simulink model "SlidingModeRobot_before_feedforard"  (R2015b)
settings: Solver=ode4  StartTime=0.0  StopTime=20  FixedStep=0.01  RelTol=1e-3
InitFcn:
  | Set_Parameter
values from neighbouring files (symbols this model uses):
  b = 0.1    [Set_Parameter_Single.m]
  J = [0.016,0.016,0.012,0.012,0.01,0.01,0.01]    [Set_Parameter_Single.m]
  K = 0.01    [Set_Parameter_Single.m]
  L = 0.5    [Set_Parameter_Single.m]
  R = 1    [Set_Parameter_Single.m]
undefined symbols (not defined in the file or in its folder): IniJointAngle
libraries: simulink x14
settings Model: Creator=User  LastModifiedBy=User

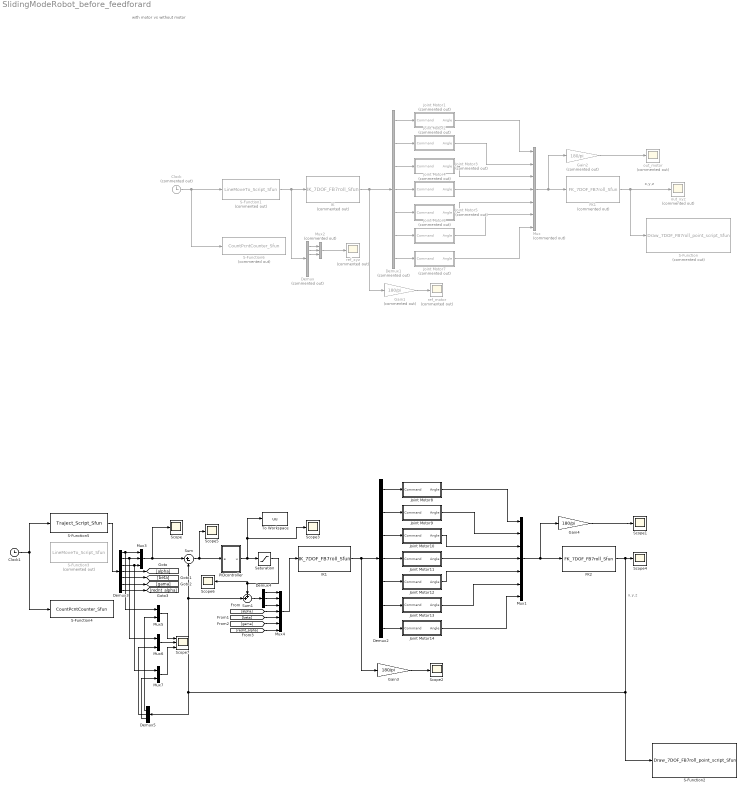
== system SlidingModeRobot_before_feedforard ==
  note: with motor vs without motor
  note: x,y,z
  note: x,y,z
  Clock : Clock  Commented=on
  Clock1 : Clock
  Demux : Demux  Commented=on  Outputs=7
  Demux1 : Demux  Commented=on  Outputs=7
  Demux2 : Demux  Outputs=7
  Demux3 : Demux  Outputs=7
  Demux4 : Demux  Outputs=3
  Demux5 : Demux  Outputs=3
  FK1 : S-Function  Commented=on  FunctionName=FK_7DOF_FB7roll_Sfun  SFunctionDeploymentMode=off  EnableBusSupport=off
  FK2 : S-Function  FunctionName=FK_7DOF_FB7roll_Sfun  SFunctionDeploymentMode=off  EnableBusSupport=off
  Gain1 : Gain  Commented=on  Gain=180/pi
  Gain2 : Gain  Commented=on  Gain=180/pi
  Gain3 : Gain  Gain=180/pi
  Gain4 : Gain  Gain=180/pi
  IK : S-Function  Commented=on  FunctionName=IK_7DOF_FB7roll_Sfun  SFunctionDeploymentMode=off  EnableBusSupport=off
  IK1 : S-Function  FunctionName=IK_7DOF_FB7roll_Sfun  SFunctionDeploymentMode=off  EnableBusSupport=off
  Joint Motor1 : Subsystem  Commented=on
  Joint Motor10 : Subsystem
  Joint Motor11 : Subsystem
  Joint Motor12 : Subsystem
  Joint Motor13 : Subsystem
  Joint Motor14 : Subsystem
  Joint Motor2 : Subsystem  Commented=on
  Joint Motor3 : Subsystem  Commented=on
  Joint Motor4 : Subsystem  Commented=on
  Joint Motor5 : Subsystem  Commented=on
  Joint Motor6 : Subsystem  Commented=on
  Joint Motor7 : Subsystem  Commented=on
  Joint Motor8 : Subsystem
  Joint Motor9 : Subsystem
  Mux : Mux  Commented=on  Inputs=7
  Mux1 : Mux  Inputs=7
  Mux2 : Mux  Commented=on  Inputs=3
  Mux3 : Mux  Inputs=3
  Mux4 : Mux  Inputs=7
  Mux5 : Mux  Inputs=2
  Mux6 : Mux  Inputs=2
  Mux7 : Mux  Inputs=2
  PIDcontroller : Subsystem
  S-Function : S-Function  Commented=on  FunctionName=Draw_7DOF_FB7roll_point_script_Sfun  SFunctionDeploymentMode=off  EnableBusSupport=off
  S-Function1 : S-Function  Commented=on  FunctionName=LineMoveTo_Script_Sfun  SFunctionDeploymentMode=off  EnableBusSupport=off
  S-Function2 : S-Function  FunctionName=Draw_7DOF_FB7roll_point_script_Sfun  SFunctionDeploymentMode=off  EnableBusSupport=off
  S-Function3 : S-Function  Commented=on  FunctionName=LineMoveTo_Script_Sfun  SFunctionDeploymentMode=off  EnableBusSupport=off
  S-Function4 : S-Function  FunctionName=CountPcntCounter_Sfun  SFunctionDeploymentMode=off  EnableBusSupport=off
  S-Function5 : S-Function  FunctionName=Traject_Script_Sfun  SFunctionDeploymentMode=off  EnableBusSupport=off
  S-Function6 : S-Function  Commented=on  FunctionName=CountPcntCounter_Sfun  SFunctionDeploymentMode=off  EnableBusSupport=off
  Saturation : Saturate  UpperLimit=50  LowerLimit=-50
  Scope{,1..6} (7 alike) : Scope
  Scope7 : Scope  NumInputPorts=3
  Sum : Sum  Inputs=|+-
  Sum1 : Sum  Inputs=++|
  To Workspace : ToWorkspace  VariableName=uu  SaveFormat=Timeseries  SampleTime=-1
  out_motor : Scope  Commented=on
  out_xyz : Scope  Commented=on
  ref_motor : Scope  Commented=on
  ref_xyz : Scope  Commented=on
  wires:
  Joint Motor3/1(Angle) -> Mux/3
  Joint Motor1/1(Angle) -> Mux/1
  Joint Motor2/1(Angle) -> Mux/2
  Joint Motor4/1(Angle) -> Mux/4
  Joint Motor5/1(Angle) -> Mux/5
  Joint Motor6/1(Angle) -> Mux/6
  Joint Motor7/1(Angle) -> Mux/7
  S-Function1/1 -> Demux/1, IK/1
  Gain1/1 -> ref_motor/1
  FK1/1 -> S-Function/1, out_xyz/1
  Gain2/1 -> out_motor/1
  Demux1/7 -> Joint Motor7/1(Command)
  Demux1/6 -> Joint Motor6/1(Command)
  Demux1/5 -> Joint Motor5/1(Command)
  Demux1/4 -> Joint Motor4/1(Command)
  Demux1/1 -> Joint Motor1/1(Command)
  Demux1/2 -> Joint Motor2/1(Command)
  Demux1/3 -> Joint Motor3/1(Command)
  IK/1 -> Demux1/1, Gain1/1
  Clock/1 -> S-Function6/1, S-Function1/1
  Mux/1 -> Gain2/1, FK1/1
  Joint Motor10/1(Angle) -> Mux1/3
  Joint Motor8/1(Angle) -> Mux1/1
  Joint Motor9/1(Angle) -> Mux1/2
  Joint Motor11/1(Angle) -> Mux1/4
  Joint Motor12/1(Angle) -> Mux1/5
  Joint Motor13/1(Angle) -> Mux1/6
  Joint Motor14/1(Angle) -> Mux1/7
  Gain3/1 -> Scope2/1
  FK2/1 -> Scope4/1, S-Function2/1, Sum1/2, Sum/2, Demux5/1
  Gain4/1 -> Scope1/1
  Demux2/7 -> Joint Motor14/1(Command)
  Demux2/6 -> Joint Motor13/1(Command)
  Demux2/5 -> Joint Motor12/1(Command)
  Demux2/4 -> Joint Motor11/1(Command)
  Demux2/1 -> Joint Motor8/1(Command)
  Demux2/2 -> Joint Motor9/1(Command)
  Demux2/3 -> Joint Motor10/1(Command)
  IK1/1 -> Demux2/1, Gain3/1
  Clock1/1 -> S-Function5/1, S-Function4/1
  Mux1/1 -> Gain4/1, FK2/1
  Sum/1 -> Scope5/1, PIDcontroller/1(e)
  Demux/1 -> Mux2/1
  Demux/2 -> Mux2/2
  Demux/3 -> Mux2/3
  Mux2/1 -> ref_xyz/1
  Demux3/1 -> Mux3/1, Mux5/1
  Demux3/2 -> Mux3/2, Mux6/1
  Demux3/3 -> Mux7/1, Mux3/3
  Demux3/4 -> [alpha]
  Demux3/5 -> [beta]
  Demux3/6 -> [gama]
  [gama] -> Mux4/6
  [beta] -> Mux4/5
  [alpha] -> Mux4/4
  Demux4/1 -> Mux4/1
  Demux4/2 -> Mux4/2
  Demux4/3 -> Mux4/3
  PIDcontroller/1(u) -> Scope3/1, To Workspace/1, Saturation/1
  Mux4/1 -> IK1/1
  Demux3/7 -> [rednt_alpha]
  [rednt_alpha] -> Mux4/7
  Sum1/1 -> Demux4/1
  Saturation/1 -> Scope6/1, Sum1/1
  S-Function5/1 -> Demux3/1
  Mux3/1 -> Sum/1, Scope/1
  Demux5/1 -> Mux5/2
  Demux5/2 -> Mux6/2
  Demux5/3 -> Mux7/2
  Mux6/1 -> Scope7/2
  Mux5/1 -> Scope7/1
  Mux7/1 -> Scope7/3

== system SlidingModeRobot_before_feedforard/Joint Motor1 ==
  Command : Inport
  Constant : Constant  Value=IniJointAngle(1)
  DC motor : Subsystem
  Gain : Gain  Gain=30
  Integrator : Integrator  InitialConditionSource=external
  PID Controller : simulink/Continuous/PID Controller  Controller=PID  TimeDomain=Continuous-time  SampleTime=-1  IntegratorMethod=Forward Euler  FilterMethod=Forward Euler  Form=Parallel  UseFilter=on  ControllerParametersSource=internal  P=20  I=0  D=20  N=0  InitialConditionSource=internal  InitialConditionForIntegrator=0  InitialConditionForFilter=0  ExternalReset=none  LimitOutput=off  UpperSaturationLimit=inf  LowerSaturationLimit=-inf  LinearizeAsGain=on  AntiWindupMode=none  Kb=1  TrackingMode=off  Kt=1  PParamMin=[]  PParamMax=[]  IParamMin=[]  IParamMax=[]  DParamMin=[]  DParamMax=[]  NParamMin=[]  NParamMax=[]  KbParamMin=[]  KbParamMax=[]  KtParamMin=[]  KtParamMax=[]  POutMin=[]  POutMax=[]  IOutMin=[]  IOutMax=[]  DOutMin=[]  DOutMax=[]  NOutMin=[]  NOutMax=[]  KbOutMin=[]  KbOutMax=[]  KtOutMin=[]  KtOutMax=[]  IntegratorOutMin=[]  IntegratorOutMax=[]  FilterOutMin=[]  FilterOutMax=[]  SumOutMin=[]  SumOutMax=[]  SumI1OutMin=[]  SumI1OutMax=[]  SumI2OutMin=[]  SumI2OutMax=[]  SumI3OutMin=[]  SumI3OutMax=[]  SumDOutMin=[]  SumDOutMax=[]  SaturationOutMin=[]  SaturationOutMax=[]  IntegratorContinuousStateAttributes=''  IntegratorStateMustResolveToSignalObject=off  IntegratorRTWStateStorageClass=Auto  FilterContinuousStateAttributes=''  FilterStateMustResolveToSignalObject=off  FilterRTWStateStorageClass=Auto  DifferentiatorICPrevScaledInput=0  DifferentiatorOutMin=[]  DifferentiatorOutMax=[]
  Sum : Sum  Inputs=|+-
  Sum1 : Sum  Inputs=|+-
  Angle : Outport
  wires:
  Sum/1 -> PID Controller/1
  PID Controller/1 -> DC motor/1(Voltage)
  DC motor/1(Speed) -> Sum/2, Integrator/1
  Integrator/1 -> Angle/1, Sum1/2
  Command/1 -> Sum1/1
  Sum1/1 -> Gain/1
  Gain/1 -> Sum/1
  Constant/1 -> Integrator/2

== system SlidingModeRobot_before_feedforard/Joint Motor10 ==
  Command : Inport
  Constant : Constant  Value=IniJointAngle(3)
  DC motor : Subsystem
  Gain : Gain  Gain=2
  Integrator : Integrator  InitialConditionSource=external
  PID Controller : simulink/Continuous/PID Controller  Controller=PID  TimeDomain=Continuous-time  SampleTime=-1  IntegratorMethod=Forward Euler  FilterMethod=Forward Euler  Form=Parallel  UseFilter=on  ControllerParametersSource=internal  P=20  I=0  D=20  N=0  InitialConditionSource=internal  InitialConditionForIntegrator=0  InitialConditionForFilter=0  ExternalReset=none  LimitOutput=off  UpperSaturationLimit=inf  LowerSaturationLimit=-inf  LinearizeAsGain=on  AntiWindupMode=none  Kb=1  TrackingMode=off  Kt=1  PParamMin=[]  PParamMax=[]  IParamMin=[]  IParamMax=[]  DParamMin=[]  DParamMax=[]  NParamMin=[]  NParamMax=[]  KbParamMin=[]  KbParamMax=[]  KtParamMin=[]  KtParamMax=[]  POutMin=[]  POutMax=[]  IOutMin=[]  IOutMax=[]  DOutMin=[]  DOutMax=[]  NOutMin=[]  NOutMax=[]  KbOutMin=[]  KbOutMax=[]  KtOutMin=[]  KtOutMax=[]  IntegratorOutMin=[]  IntegratorOutMax=[]  FilterOutMin=[]  FilterOutMax=[]  SumOutMin=[]  SumOutMax=[]  SumI1OutMin=[]  SumI1OutMax=[]  SumI2OutMin=[]  SumI2OutMax=[]  SumI3OutMin=[]  SumI3OutMax=[]  SumDOutMin=[]  SumDOutMax=[]  SaturationOutMin=[]  SaturationOutMax=[]  IntegratorContinuousStateAttributes=''  IntegratorStateMustResolveToSignalObject=off  IntegratorRTWStateStorageClass=Auto  FilterContinuousStateAttributes=''  FilterStateMustResolveToSignalObject=off  FilterRTWStateStorageClass=Auto  DifferentiatorICPrevScaledInput=0  DifferentiatorOutMin=[]  DifferentiatorOutMax=[]
  Sum : Sum  Inputs=|+-
  Sum1 : Sum  Inputs=|+-
  Angle : Outport
  wires:
  Sum/1 -> PID Controller/1
  PID Controller/1 -> DC motor/1(Voltage)
  DC motor/1(Speed) -> Sum/2, Integrator/1
  Integrator/1 -> Angle/1, Sum1/2
  Command/1 -> Sum1/1
  Sum1/1 -> Gain/1
  Gain/1 -> Sum/1
  Constant/1 -> Integrator/2

== system SlidingModeRobot_before_feedforard/Joint Motor11 ==
  Command : Inport
  Constant : Constant  Value=IniJointAngle(4)
  DC motor : Subsystem
  Gain : Gain  Gain=2
  Integrator : Integrator  InitialConditionSource=external
  PID Controller : simulink/Continuous/PID Controller  Controller=PID  TimeDomain=Continuous-time  SampleTime=-1  IntegratorMethod=Forward Euler  FilterMethod=Forward Euler  Form=Parallel  UseFilter=on  ControllerParametersSource=internal  P=20  I=0  D=20  N=0  InitialConditionSource=internal  InitialConditionForIntegrator=0  InitialConditionForFilter=0  ExternalReset=none  LimitOutput=off  UpperSaturationLimit=inf  LowerSaturationLimit=-inf  LinearizeAsGain=on  AntiWindupMode=none  Kb=1  TrackingMode=off  Kt=1  PParamMin=[]  PParamMax=[]  IParamMin=[]  IParamMax=[]  DParamMin=[]  DParamMax=[]  NParamMin=[]  NParamMax=[]  KbParamMin=[]  KbParamMax=[]  KtParamMin=[]  KtParamMax=[]  POutMin=[]  POutMax=[]  IOutMin=[]  IOutMax=[]  DOutMin=[]  DOutMax=[]  NOutMin=[]  NOutMax=[]  KbOutMin=[]  KbOutMax=[]  KtOutMin=[]  KtOutMax=[]  IntegratorOutMin=[]  IntegratorOutMax=[]  FilterOutMin=[]  FilterOutMax=[]  SumOutMin=[]  SumOutMax=[]  SumI1OutMin=[]  SumI1OutMax=[]  SumI2OutMin=[]  SumI2OutMax=[]  SumI3OutMin=[]  SumI3OutMax=[]  SumDOutMin=[]  SumDOutMax=[]  SaturationOutMin=[]  SaturationOutMax=[]  IntegratorContinuousStateAttributes=''  IntegratorStateMustResolveToSignalObject=off  IntegratorRTWStateStorageClass=Auto  FilterContinuousStateAttributes=''  FilterStateMustResolveToSignalObject=off  FilterRTWStateStorageClass=Auto  DifferentiatorICPrevScaledInput=0  DifferentiatorOutMin=[]  DifferentiatorOutMax=[]
  Sum : Sum  Inputs=|+-
  Sum1 : Sum  Inputs=|+-
  Angle : Outport
  wires:
  Sum/1 -> PID Controller/1
  PID Controller/1 -> DC motor/1(Voltage)
  DC motor/1(Speed) -> Sum/2, Integrator/1
  Integrator/1 -> Angle/1, Sum1/2
  Command/1 -> Sum1/1
  Sum1/1 -> Gain/1
  Gain/1 -> Sum/1
  Constant/1 -> Integrator/2

== system SlidingModeRobot_before_feedforard/Joint Motor12 ==
  Command : Inport
  Constant : Constant  Value=IniJointAngle(5)
  DC motor : Subsystem
  Gain : Gain  Gain=2
  Integrator : Integrator  InitialConditionSource=external
  PID Controller : simulink/Continuous/PID Controller  Controller=PID  TimeDomain=Continuous-time  SampleTime=-1  IntegratorMethod=Forward Euler  FilterMethod=Forward Euler  Form=Parallel  UseFilter=on  ControllerParametersSource=internal  P=20  I=0  D=20  N=0  InitialConditionSource=internal  InitialConditionForIntegrator=0  InitialConditionForFilter=0  ExternalReset=none  LimitOutput=off  UpperSaturationLimit=inf  LowerSaturationLimit=-inf  LinearizeAsGain=on  AntiWindupMode=none  Kb=1  TrackingMode=off  Kt=1  PParamMin=[]  PParamMax=[]  IParamMin=[]  IParamMax=[]  DParamMin=[]  DParamMax=[]  NParamMin=[]  NParamMax=[]  KbParamMin=[]  KbParamMax=[]  KtParamMin=[]  KtParamMax=[]  POutMin=[]  POutMax=[]  IOutMin=[]  IOutMax=[]  DOutMin=[]  DOutMax=[]  NOutMin=[]  NOutMax=[]  KbOutMin=[]  KbOutMax=[]  KtOutMin=[]  KtOutMax=[]  IntegratorOutMin=[]  IntegratorOutMax=[]  FilterOutMin=[]  FilterOutMax=[]  SumOutMin=[]  SumOutMax=[]  SumI1OutMin=[]  SumI1OutMax=[]  SumI2OutMin=[]  SumI2OutMax=[]  SumI3OutMin=[]  SumI3OutMax=[]  SumDOutMin=[]  SumDOutMax=[]  SaturationOutMin=[]  SaturationOutMax=[]  IntegratorContinuousStateAttributes=''  IntegratorStateMustResolveToSignalObject=off  IntegratorRTWStateStorageClass=Auto  FilterContinuousStateAttributes=''  FilterStateMustResolveToSignalObject=off  FilterRTWStateStorageClass=Auto  DifferentiatorICPrevScaledInput=0  DifferentiatorOutMin=[]  DifferentiatorOutMax=[]
  Sum : Sum  Inputs=|+-
  Sum1 : Sum  Inputs=|+-
  Angle : Outport
  wires:
  Sum/1 -> PID Controller/1
  PID Controller/1 -> DC motor/1(Voltage)
  DC motor/1(Speed) -> Sum/2, Integrator/1
  Integrator/1 -> Angle/1, Sum1/2
  Command/1 -> Sum1/1
  Sum1/1 -> Gain/1
  Gain/1 -> Sum/1
  Constant/1 -> Integrator/2

== system SlidingModeRobot_before_feedforard/Joint Motor13 ==
  Command : Inport
  Constant : Constant  Value=IniJointAngle(6)
  DC motor : Subsystem
  Gain : Gain  Gain=2
  Integrator : Integrator  InitialConditionSource=external
  PID Controller : simulink/Continuous/PID Controller  Controller=PID  TimeDomain=Continuous-time  SampleTime=-1  IntegratorMethod=Forward Euler  FilterMethod=Forward Euler  Form=Parallel  UseFilter=on  ControllerParametersSource=internal  P=20  I=0  D=20  N=0  InitialConditionSource=internal  InitialConditionForIntegrator=0  InitialConditionForFilter=0  ExternalReset=none  LimitOutput=off  UpperSaturationLimit=inf  LowerSaturationLimit=-inf  LinearizeAsGain=on  AntiWindupMode=none  Kb=1  TrackingMode=off  Kt=1  PParamMin=[]  PParamMax=[]  IParamMin=[]  IParamMax=[]  DParamMin=[]  DParamMax=[]  NParamMin=[]  NParamMax=[]  KbParamMin=[]  KbParamMax=[]  KtParamMin=[]  KtParamMax=[]  POutMin=[]  POutMax=[]  IOutMin=[]  IOutMax=[]  DOutMin=[]  DOutMax=[]  NOutMin=[]  NOutMax=[]  KbOutMin=[]  KbOutMax=[]  KtOutMin=[]  KtOutMax=[]  IntegratorOutMin=[]  IntegratorOutMax=[]  FilterOutMin=[]  FilterOutMax=[]  SumOutMin=[]  SumOutMax=[]  SumI1OutMin=[]  SumI1OutMax=[]  SumI2OutMin=[]  SumI2OutMax=[]  SumI3OutMin=[]  SumI3OutMax=[]  SumDOutMin=[]  SumDOutMax=[]  SaturationOutMin=[]  SaturationOutMax=[]  IntegratorContinuousStateAttributes=''  IntegratorStateMustResolveToSignalObject=off  IntegratorRTWStateStorageClass=Auto  FilterContinuousStateAttributes=''  FilterStateMustResolveToSignalObject=off  FilterRTWStateStorageClass=Auto  DifferentiatorICPrevScaledInput=0  DifferentiatorOutMin=[]  DifferentiatorOutMax=[]
  Sum : Sum  Inputs=|+-
  Sum1 : Sum  Inputs=|+-
  Angle : Outport
  wires:
  Sum/1 -> PID Controller/1
  PID Controller/1 -> DC motor/1(Voltage)
  DC motor/1(Speed) -> Sum/2, Integrator/1
  Integrator/1 -> Angle/1, Sum1/2
  Command/1 -> Sum1/1
  Sum1/1 -> Gain/1
  Gain/1 -> Sum/1
  Constant/1 -> Integrator/2

== system SlidingModeRobot_before_feedforard/Joint Motor14 ==
  Command : Inport
  Constant : Constant  Value=IniJointAngle(7)
  DC motor : Subsystem
  Gain : Gain  Gain=2
  Integrator : Integrator  InitialConditionSource=external
  PID Controller : simulink/Continuous/PID Controller  Controller=PID  TimeDomain=Continuous-time  SampleTime=-1  IntegratorMethod=Forward Euler  FilterMethod=Forward Euler  Form=Parallel  UseFilter=on  ControllerParametersSource=internal  P=20  I=0  D=20  N=0  InitialConditionSource=internal  InitialConditionForIntegrator=0  InitialConditionForFilter=0  ExternalReset=none  LimitOutput=off  UpperSaturationLimit=inf  LowerSaturationLimit=-inf  LinearizeAsGain=on  AntiWindupMode=none  Kb=1  TrackingMode=off  Kt=1  PParamMin=[]  PParamMax=[]  IParamMin=[]  IParamMax=[]  DParamMin=[]  DParamMax=[]  NParamMin=[]  NParamMax=[]  KbParamMin=[]  KbParamMax=[]  KtParamMin=[]  KtParamMax=[]  POutMin=[]  POutMax=[]  IOutMin=[]  IOutMax=[]  DOutMin=[]  DOutMax=[]  NOutMin=[]  NOutMax=[]  KbOutMin=[]  KbOutMax=[]  KtOutMin=[]  KtOutMax=[]  IntegratorOutMin=[]  IntegratorOutMax=[]  FilterOutMin=[]  FilterOutMax=[]  SumOutMin=[]  SumOutMax=[]  SumI1OutMin=[]  SumI1OutMax=[]  SumI2OutMin=[]  SumI2OutMax=[]  SumI3OutMin=[]  SumI3OutMax=[]  SumDOutMin=[]  SumDOutMax=[]  SaturationOutMin=[]  SaturationOutMax=[]  IntegratorContinuousStateAttributes=''  IntegratorStateMustResolveToSignalObject=off  IntegratorRTWStateStorageClass=Auto  FilterContinuousStateAttributes=''  FilterStateMustResolveToSignalObject=off  FilterRTWStateStorageClass=Auto  DifferentiatorICPrevScaledInput=0  DifferentiatorOutMin=[]  DifferentiatorOutMax=[]
  Sum : Sum  Inputs=|+-
  Sum1 : Sum  Inputs=|+-
  Angle : Outport
  wires:
  Sum/1 -> PID Controller/1
  PID Controller/1 -> DC motor/1(Voltage)
  DC motor/1(Speed) -> Sum/2, Integrator/1
  Integrator/1 -> Angle/1, Sum1/2
  Command/1 -> Sum1/1
  Sum1/1 -> Gain/1
  Gain/1 -> Sum/1
  Constant/1 -> Integrator/2

== system SlidingModeRobot_before_feedforard/Joint Motor2 ==
  Command : Inport
  Constant : Constant  Value=IniJointAngle(2)
  DC motor : Subsystem
  Gain : Gain  Gain=32
  Integrator : Integrator  InitialConditionSource=external
  PID Controller : simulink/Continuous/PID Controller  Controller=PID  TimeDomain=Continuous-time  SampleTime=-1  IntegratorMethod=Forward Euler  FilterMethod=Forward Euler  Form=Parallel  UseFilter=on  ControllerParametersSource=internal  P=20  I=0  D=20  N=0  InitialConditionSource=internal  InitialConditionForIntegrator=0  InitialConditionForFilter=0  ExternalReset=none  LimitOutput=off  UpperSaturationLimit=inf  LowerSaturationLimit=-inf  LinearizeAsGain=on  AntiWindupMode=none  Kb=1  TrackingMode=off  Kt=1  PParamMin=[]  PParamMax=[]  IParamMin=[]  IParamMax=[]  DParamMin=[]  DParamMax=[]  NParamMin=[]  NParamMax=[]  KbParamMin=[]  KbParamMax=[]  KtParamMin=[]  KtParamMax=[]  POutMin=[]  POutMax=[]  IOutMin=[]  IOutMax=[]  DOutMin=[]  DOutMax=[]  NOutMin=[]  NOutMax=[]  KbOutMin=[]  KbOutMax=[]  KtOutMin=[]  KtOutMax=[]  IntegratorOutMin=[]  IntegratorOutMax=[]  FilterOutMin=[]  FilterOutMax=[]  SumOutMin=[]  SumOutMax=[]  SumI1OutMin=[]  SumI1OutMax=[]  SumI2OutMin=[]  SumI2OutMax=[]  SumI3OutMin=[]  SumI3OutMax=[]  SumDOutMin=[]  SumDOutMax=[]  SaturationOutMin=[]  SaturationOutMax=[]  IntegratorContinuousStateAttributes=''  IntegratorStateMustResolveToSignalObject=off  IntegratorRTWStateStorageClass=Auto  FilterContinuousStateAttributes=''  FilterStateMustResolveToSignalObject=off  FilterRTWStateStorageClass=Auto  DifferentiatorICPrevScaledInput=0  DifferentiatorOutMin=[]  DifferentiatorOutMax=[]
  Sum : Sum  Inputs=|+-
  Sum1 : Sum  Inputs=|+-
  Angle : Outport
  wires:
  Sum/1 -> PID Controller/1
  PID Controller/1 -> DC motor/1(Voltage)
  DC motor/1(Speed) -> Sum/2, Integrator/1
  Integrator/1 -> Angle/1, Sum1/2
  Command/1 -> Sum1/1
  Sum1/1 -> Gain/1
  Gain/1 -> Sum/1
  Constant/1 -> Integrator/2

== system SlidingModeRobot_before_feedforard/Joint Motor3 ==
  Command : Inport
  Constant : Constant  Value=IniJointAngle(3)
  DC motor : Subsystem
  Gain : Gain  Gain=30
  Integrator : Integrator  InitialConditionSource=external
  PID Controller : simulink/Continuous/PID Controller  Controller=PID  TimeDomain=Continuous-time  SampleTime=-1  IntegratorMethod=Forward Euler  FilterMethod=Forward Euler  Form=Parallel  UseFilter=on  ControllerParametersSource=internal  P=20  I=0  D=20  N=0  InitialConditionSource=internal  InitialConditionForIntegrator=0  InitialConditionForFilter=0  ExternalReset=none  LimitOutput=off  UpperSaturationLimit=inf  LowerSaturationLimit=-inf  LinearizeAsGain=on  AntiWindupMode=none  Kb=1  TrackingMode=off  Kt=1  PParamMin=[]  PParamMax=[]  IParamMin=[]  IParamMax=[]  DParamMin=[]  DParamMax=[]  NParamMin=[]  NParamMax=[]  KbParamMin=[]  KbParamMax=[]  KtParamMin=[]  KtParamMax=[]  POutMin=[]  POutMax=[]  IOutMin=[]  IOutMax=[]  DOutMin=[]  DOutMax=[]  NOutMin=[]  NOutMax=[]  KbOutMin=[]  KbOutMax=[]  KtOutMin=[]  KtOutMax=[]  IntegratorOutMin=[]  IntegratorOutMax=[]  FilterOutMin=[]  FilterOutMax=[]  SumOutMin=[]  SumOutMax=[]  SumI1OutMin=[]  SumI1OutMax=[]  SumI2OutMin=[]  SumI2OutMax=[]  SumI3OutMin=[]  SumI3OutMax=[]  SumDOutMin=[]  SumDOutMax=[]  SaturationOutMin=[]  SaturationOutMax=[]  IntegratorContinuousStateAttributes=''  IntegratorStateMustResolveToSignalObject=off  IntegratorRTWStateStorageClass=Auto  FilterContinuousStateAttributes=''  FilterStateMustResolveToSignalObject=off  FilterRTWStateStorageClass=Auto  DifferentiatorICPrevScaledInput=0  DifferentiatorOutMin=[]  DifferentiatorOutMax=[]
  Sum : Sum  Inputs=|+-
  Sum1 : Sum  Inputs=|+-
  Angle : Outport
  wires:
  Sum/1 -> PID Controller/1
  PID Controller/1 -> DC motor/1(Voltage)
  DC motor/1(Speed) -> Sum/2, Integrator/1
  Integrator/1 -> Angle/1, Sum1/2
  Command/1 -> Sum1/1
  Sum1/1 -> Gain/1
  Gain/1 -> Sum/1
  Constant/1 -> Integrator/2

== system SlidingModeRobot_before_feedforard/Joint Motor4 ==
  Command : Inport
  Constant : Constant  Value=IniJointAngle(4)
  DC motor : Subsystem
  Gain : Gain  Gain=10
  Integrator : Integrator  InitialConditionSource=external
  PID Controller : simulink/Continuous/PID Controller  Controller=PID  TimeDomain=Continuous-time  SampleTime=-1  IntegratorMethod=Forward Euler  FilterMethod=Forward Euler  Form=Parallel  UseFilter=on  ControllerParametersSource=internal  P=20  I=0  D=20  N=0  InitialConditionSource=internal  InitialConditionForIntegrator=0  InitialConditionForFilter=0  ExternalReset=none  LimitOutput=off  UpperSaturationLimit=inf  LowerSaturationLimit=-inf  LinearizeAsGain=on  AntiWindupMode=none  Kb=1  TrackingMode=off  Kt=1  PParamMin=[]  PParamMax=[]  IParamMin=[]  IParamMax=[]  DParamMin=[]  DParamMax=[]  NParamMin=[]  NParamMax=[]  KbParamMin=[]  KbParamMax=[]  KtParamMin=[]  KtParamMax=[]  POutMin=[]  POutMax=[]  IOutMin=[]  IOutMax=[]  DOutMin=[]  DOutMax=[]  NOutMin=[]  NOutMax=[]  KbOutMin=[]  KbOutMax=[]  KtOutMin=[]  KtOutMax=[]  IntegratorOutMin=[]  IntegratorOutMax=[]  FilterOutMin=[]  FilterOutMax=[]  SumOutMin=[]  SumOutMax=[]  SumI1OutMin=[]  SumI1OutMax=[]  SumI2OutMin=[]  SumI2OutMax=[]  SumI3OutMin=[]  SumI3OutMax=[]  SumDOutMin=[]  SumDOutMax=[]  SaturationOutMin=[]  SaturationOutMax=[]  IntegratorContinuousStateAttributes=''  IntegratorStateMustResolveToSignalObject=off  IntegratorRTWStateStorageClass=Auto  FilterContinuousStateAttributes=''  FilterStateMustResolveToSignalObject=off  FilterRTWStateStorageClass=Auto  DifferentiatorICPrevScaledInput=0  DifferentiatorOutMin=[]  DifferentiatorOutMax=[]
  Sum : Sum  Inputs=|+-
  Sum1 : Sum  Inputs=|+-
  Angle : Outport
  wires:
  Sum/1 -> PID Controller/1
  PID Controller/1 -> DC motor/1(Voltage)
  DC motor/1(Speed) -> Sum/2, Integrator/1
  Integrator/1 -> Angle/1, Sum1/2
  Command/1 -> Sum1/1
  Sum1/1 -> Gain/1
  Gain/1 -> Sum/1
  Constant/1 -> Integrator/2

== system SlidingModeRobot_before_feedforard/Joint Motor5 ==
  Command : Inport
  Constant : Constant  Value=IniJointAngle(5)
  DC motor : Subsystem
  Gain : Gain  Gain=2
  Integrator : Integrator  InitialConditionSource=external
  PID Controller : simulink/Continuous/PID Controller  Controller=PID  TimeDomain=Continuous-time  SampleTime=-1  IntegratorMethod=Forward Euler  FilterMethod=Forward Euler  Form=Parallel  UseFilter=on  ControllerParametersSource=internal  P=20  I=0  D=20  N=0  InitialConditionSource=internal  InitialConditionForIntegrator=0  InitialConditionForFilter=0  ExternalReset=none  LimitOutput=off  UpperSaturationLimit=inf  LowerSaturationLimit=-inf  LinearizeAsGain=on  AntiWindupMode=none  Kb=1  TrackingMode=off  Kt=1  PParamMin=[]  PParamMax=[]  IParamMin=[]  IParamMax=[]  DParamMin=[]  DParamMax=[]  NParamMin=[]  NParamMax=[]  KbParamMin=[]  KbParamMax=[]  KtParamMin=[]  KtParamMax=[]  POutMin=[]  POutMax=[]  IOutMin=[]  IOutMax=[]  DOutMin=[]  DOutMax=[]  NOutMin=[]  NOutMax=[]  KbOutMin=[]  KbOutMax=[]  KtOutMin=[]  KtOutMax=[]  IntegratorOutMin=[]  IntegratorOutMax=[]  FilterOutMin=[]  FilterOutMax=[]  SumOutMin=[]  SumOutMax=[]  SumI1OutMin=[]  SumI1OutMax=[]  SumI2OutMin=[]  SumI2OutMax=[]  SumI3OutMin=[]  SumI3OutMax=[]  SumDOutMin=[]  SumDOutMax=[]  SaturationOutMin=[]  SaturationOutMax=[]  IntegratorContinuousStateAttributes=''  IntegratorStateMustResolveToSignalObject=off  IntegratorRTWStateStorageClass=Auto  FilterContinuousStateAttributes=''  FilterStateMustResolveToSignalObject=off  FilterRTWStateStorageClass=Auto  DifferentiatorICPrevScaledInput=0  DifferentiatorOutMin=[]  DifferentiatorOutMax=[]
  Sum : Sum  Inputs=|+-
  Sum1 : Sum  Inputs=|+-
  Angle : Outport
  wires:
  Sum/1 -> PID Controller/1
  PID Controller/1 -> DC motor/1(Voltage)
  DC motor/1(Speed) -> Sum/2, Integrator/1
  Integrator/1 -> Angle/1, Sum1/2
  Command/1 -> Sum1/1
  Sum1/1 -> Gain/1
  Gain/1 -> Sum/1
  Constant/1 -> Integrator/2

== system SlidingModeRobot_before_feedforard/Joint Motor6 ==
  Command : Inport
  Constant : Constant  Value=IniJointAngle(6)
  DC motor : Subsystem
  Gain : Gain  Gain=2
  Integrator : Integrator  InitialConditionSource=external
  PID Controller : simulink/Continuous/PID Controller  Controller=PID  TimeDomain=Continuous-time  SampleTime=-1  IntegratorMethod=Forward Euler  FilterMethod=Forward Euler  Form=Parallel  UseFilter=on  ControllerParametersSource=internal  P=20  I=0  D=20  N=0  InitialConditionSource=internal  InitialConditionForIntegrator=0  InitialConditionForFilter=0  ExternalReset=none  LimitOutput=off  UpperSaturationLimit=inf  LowerSaturationLimit=-inf  LinearizeAsGain=on  AntiWindupMode=none  Kb=1  TrackingMode=off  Kt=1  PParamMin=[]  PParamMax=[]  IParamMin=[]  IParamMax=[]  DParamMin=[]  DParamMax=[]  NParamMin=[]  NParamMax=[]  KbParamMin=[]  KbParamMax=[]  KtParamMin=[]  KtParamMax=[]  POutMin=[]  POutMax=[]  IOutMin=[]  IOutMax=[]  DOutMin=[]  DOutMax=[]  NOutMin=[]  NOutMax=[]  KbOutMin=[]  KbOutMax=[]  KtOutMin=[]  KtOutMax=[]  IntegratorOutMin=[]  IntegratorOutMax=[]  FilterOutMin=[]  FilterOutMax=[]  SumOutMin=[]  SumOutMax=[]  SumI1OutMin=[]  SumI1OutMax=[]  SumI2OutMin=[]  SumI2OutMax=[]  SumI3OutMin=[]  SumI3OutMax=[]  SumDOutMin=[]  SumDOutMax=[]  SaturationOutMin=[]  SaturationOutMax=[]  IntegratorContinuousStateAttributes=''  IntegratorStateMustResolveToSignalObject=off  IntegratorRTWStateStorageClass=Auto  FilterContinuousStateAttributes=''  FilterStateMustResolveToSignalObject=off  FilterRTWStateStorageClass=Auto  DifferentiatorICPrevScaledInput=0  DifferentiatorOutMin=[]  DifferentiatorOutMax=[]
  Sum : Sum  Inputs=|+-
  Sum1 : Sum  Inputs=|+-
  Angle : Outport
  wires:
  Sum/1 -> PID Controller/1
  PID Controller/1 -> DC motor/1(Voltage)
  DC motor/1(Speed) -> Sum/2, Integrator/1
  Integrator/1 -> Angle/1, Sum1/2
  Command/1 -> Sum1/1
  Sum1/1 -> Gain/1
  Gain/1 -> Sum/1
  Constant/1 -> Integrator/2

== system SlidingModeRobot_before_feedforard/Joint Motor7 ==
  Command : Inport
  Constant : Constant  Value=IniJointAngle(7)
  DC motor : Subsystem
  Gain : Gain  Gain=2
  Integrator : Integrator  InitialConditionSource=external
  PID Controller : simulink/Continuous/PID Controller  Controller=PID  TimeDomain=Continuous-time  SampleTime=-1  IntegratorMethod=Forward Euler  FilterMethod=Forward Euler  Form=Parallel  UseFilter=on  ControllerParametersSource=internal  P=20  I=0  D=20  N=0  InitialConditionSource=internal  InitialConditionForIntegrator=0  InitialConditionForFilter=0  ExternalReset=none  LimitOutput=off  UpperSaturationLimit=inf  LowerSaturationLimit=-inf  LinearizeAsGain=on  AntiWindupMode=none  Kb=1  TrackingMode=off  Kt=1  PParamMin=[]  PParamMax=[]  IParamMin=[]  IParamMax=[]  DParamMin=[]  DParamMax=[]  NParamMin=[]  NParamMax=[]  KbParamMin=[]  KbParamMax=[]  KtParamMin=[]  KtParamMax=[]  POutMin=[]  POutMax=[]  IOutMin=[]  IOutMax=[]  DOutMin=[]  DOutMax=[]  NOutMin=[]  NOutMax=[]  KbOutMin=[]  KbOutMax=[]  KtOutMin=[]  KtOutMax=[]  IntegratorOutMin=[]  IntegratorOutMax=[]  FilterOutMin=[]  FilterOutMax=[]  SumOutMin=[]  SumOutMax=[]  SumI1OutMin=[]  SumI1OutMax=[]  SumI2OutMin=[]  SumI2OutMax=[]  SumI3OutMin=[]  SumI3OutMax=[]  SumDOutMin=[]  SumDOutMax=[]  SaturationOutMin=[]  SaturationOutMax=[]  IntegratorContinuousStateAttributes=''  IntegratorStateMustResolveToSignalObject=off  IntegratorRTWStateStorageClass=Auto  FilterContinuousStateAttributes=''  FilterStateMustResolveToSignalObject=off  FilterRTWStateStorageClass=Auto  DifferentiatorICPrevScaledInput=0  DifferentiatorOutMin=[]  DifferentiatorOutMax=[]
  Sum : Sum  Inputs=|+-
  Sum1 : Sum  Inputs=|+-
  Angle : Outport
  wires:
  Sum/1 -> PID Controller/1
  PID Controller/1 -> DC motor/1(Voltage)
  DC motor/1(Speed) -> Sum/2, Integrator/1
  Integrator/1 -> Angle/1, Sum1/2
  Command/1 -> Sum1/1
  Sum1/1 -> Gain/1
  Gain/1 -> Sum/1
  Constant/1 -> Integrator/2

== system SlidingModeRobot_before_feedforard/Joint Motor8 ==
  Command : Inport
  Constant : Constant  Value=IniJointAngle(1)
  DC motor : Subsystem
  Gain : Gain  Gain=2
  Integrator : Integrator  InitialConditionSource=external
  PID Controller : simulink/Continuous/PID Controller  Controller=PID  TimeDomain=Continuous-time  SampleTime=-1  IntegratorMethod=Forward Euler  FilterMethod=Forward Euler  Form=Parallel  UseFilter=on  ControllerParametersSource=internal  P=20  I=0  D=20  N=0  InitialConditionSource=internal  InitialConditionForIntegrator=0  InitialConditionForFilter=0  ExternalReset=none  LimitOutput=off  UpperSaturationLimit=inf  LowerSaturationLimit=-inf  LinearizeAsGain=on  AntiWindupMode=none  Kb=1  TrackingMode=off  Kt=1  PParamMin=[]  PParamMax=[]  IParamMin=[]  IParamMax=[]  DParamMin=[]  DParamMax=[]  NParamMin=[]  NParamMax=[]  KbParamMin=[]  KbParamMax=[]  KtParamMin=[]  KtParamMax=[]  POutMin=[]  POutMax=[]  IOutMin=[]  IOutMax=[]  DOutMin=[]  DOutMax=[]  NOutMin=[]  NOutMax=[]  KbOutMin=[]  KbOutMax=[]  KtOutMin=[]  KtOutMax=[]  IntegratorOutMin=[]  IntegratorOutMax=[]  FilterOutMin=[]  FilterOutMax=[]  SumOutMin=[]  SumOutMax=[]  SumI1OutMin=[]  SumI1OutMax=[]  SumI2OutMin=[]  SumI2OutMax=[]  SumI3OutMin=[]  SumI3OutMax=[]  SumDOutMin=[]  SumDOutMax=[]  SaturationOutMin=[]  SaturationOutMax=[]  IntegratorContinuousStateAttributes=''  IntegratorStateMustResolveToSignalObject=off  IntegratorRTWStateStorageClass=Auto  FilterContinuousStateAttributes=''  FilterStateMustResolveToSignalObject=off  FilterRTWStateStorageClass=Auto  DifferentiatorICPrevScaledInput=0  DifferentiatorOutMin=[]  DifferentiatorOutMax=[]
  Sum : Sum  Inputs=|+-
  Sum1 : Sum  Inputs=|+-
  Angle : Outport
  wires:
  Sum/1 -> PID Controller/1
  PID Controller/1 -> DC motor/1(Voltage)
  DC motor/1(Speed) -> Sum/2, Integrator/1
  Integrator/1 -> Angle/1, Sum1/2
  Command/1 -> Sum1/1
  Sum1/1 -> Gain/1
  Gain/1 -> Sum/1
  Constant/1 -> Integrator/2

== system SlidingModeRobot_before_feedforard/Joint Motor9 ==
  Command : Inport
  Constant : Constant  Value=IniJointAngle(2)
  DC motor : Subsystem
  Gain : Gain  Gain=2
  Integrator : Integrator  InitialConditionSource=external
  PID Controller : simulink/Continuous/PID Controller  Controller=PID  TimeDomain=Continuous-time  SampleTime=-1  IntegratorMethod=Forward Euler  FilterMethod=Forward Euler  Form=Parallel  UseFilter=on  ControllerParametersSource=internal  P=20  I=0  D=20  N=0  InitialConditionSource=internal  InitialConditionForIntegrator=0  InitialConditionForFilter=0  ExternalReset=none  LimitOutput=off  UpperSaturationLimit=inf  LowerSaturationLimit=-inf  LinearizeAsGain=on  AntiWindupMode=none  Kb=1  TrackingMode=off  Kt=1  PParamMin=[]  PParamMax=[]  IParamMin=[]  IParamMax=[]  DParamMin=[]  DParamMax=[]  NParamMin=[]  NParamMax=[]  KbParamMin=[]  KbParamMax=[]  KtParamMin=[]  KtParamMax=[]  POutMin=[]  POutMax=[]  IOutMin=[]  IOutMax=[]  DOutMin=[]  DOutMax=[]  NOutMin=[]  NOutMax=[]  KbOutMin=[]  KbOutMax=[]  KtOutMin=[]  KtOutMax=[]  IntegratorOutMin=[]  IntegratorOutMax=[]  FilterOutMin=[]  FilterOutMax=[]  SumOutMin=[]  SumOutMax=[]  SumI1OutMin=[]  SumI1OutMax=[]  SumI2OutMin=[]  SumI2OutMax=[]  SumI3OutMin=[]  SumI3OutMax=[]  SumDOutMin=[]  SumDOutMax=[]  SaturationOutMin=[]  SaturationOutMax=[]  IntegratorContinuousStateAttributes=''  IntegratorStateMustResolveToSignalObject=off  IntegratorRTWStateStorageClass=Auto  FilterContinuousStateAttributes=''  FilterStateMustResolveToSignalObject=off  FilterRTWStateStorageClass=Auto  DifferentiatorICPrevScaledInput=0  DifferentiatorOutMin=[]  DifferentiatorOutMax=[]
  Sum : Sum  Inputs=|+-
  Sum1 : Sum  Inputs=|+-
  Angle : Outport
  wires:
  Sum/1 -> PID Controller/1
  PID Controller/1 -> DC motor/1(Voltage)
  DC motor/1(Speed) -> Sum/2, Integrator/1
  Integrator/1 -> Angle/1, Sum1/2
  Command/1 -> Sum1/1
  Sum1/1 -> Gain/1
  Gain/1 -> Sum/1
  Constant/1 -> Integrator/2

== system SlidingModeRobot_before_feedforard/PIDcontroller ==
  e : Inport
  D gain : Gain  Gain=0.9
  D scope : Scope
  Derivative : Derivative
  I gain : Gain  Gain=1.3
  I scope : Scope
  Integrator : Integrator
  P gain : Gain  Gain=8
  P scope : Scope
  Sum1 : Sum  Inputs=+++
  u : Outport
  wires:
  I gain/1 -> Integrator/1
  P gain/1 -> P scope/1, Sum1/1
  Integrator/1 -> I scope/1, Sum1/2
  e/1 -> D gain/1, I gain/1, P gain/1
  Sum1/1 -> u/1
  D gain/1 -> Derivative/1
  Derivative/1 -> D scope/1, Sum1/3

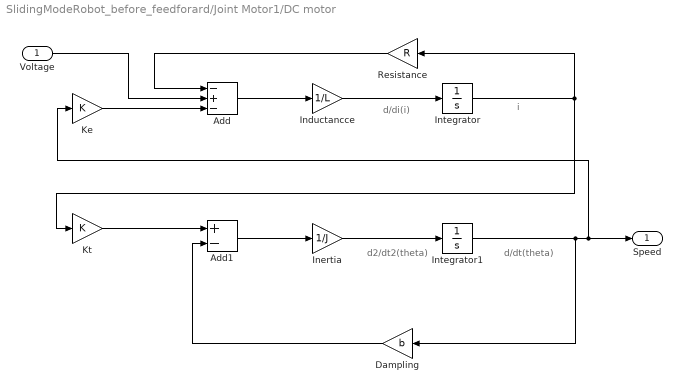
== system SlidingModeRobot_before_feedforard/Joint Motor1/DC motor ==
  note: d/dt(theta)
  note: d2/dt2(theta)
  note: i
  note: d/di(i)
  Voltage : Inport
  Add : Sum  Inputs=-+-
  Add1 : Sum  Inputs=+-
  Dampling : Gain  Gain=b
  Inductancce : Gain  Gain=1/L
  Inertia : Gain  Gain=1/J
  Integrator : Integrator
  Integrator1 : Integrator
  Ke : Gain  Gain=K
  Kt : Gain  Gain=K
  Resistance : Gain  Gain=R
  Speed : Outport
  wires:
  Resistance/1 -> Add/1
  Add/1 -> Inductancce/1
  Inductancce/1 -> Integrator/1
  Inertia/1 -> Integrator1/1
  Kt/1 -> Add1/1
  Add1/1 -> Inertia/1
  Integrator/1 -> Kt/1, Resistance/1
  Voltage/1 -> Add/2
  Dampling/1 -> Add1/2
  Integrator1/1 -> Dampling/1, Speed/1, Ke/1
  Ke/1 -> Add/3

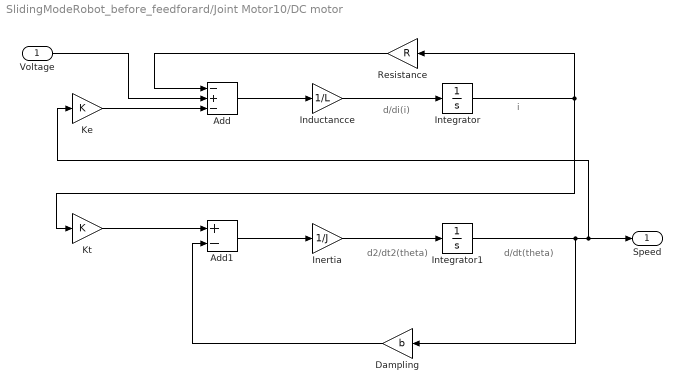
== system SlidingModeRobot_before_feedforard/Joint Motor10/DC motor ==
  note: d/dt(theta)
  note: d2/dt2(theta)
  note: i
  note: d/di(i)
  Voltage : Inport
  Add : Sum  Inputs=-+-
  Add1 : Sum  Inputs=+-
  Dampling : Gain  Gain=b
  Inductancce : Gain  Gain=1/L
  Inertia : Gain  Gain=1/J
  Integrator : Integrator
  Integrator1 : Integrator
  Ke : Gain  Gain=K
  Kt : Gain  Gain=K
  Resistance : Gain  Gain=R
  Speed : Outport
  wires:
  Resistance/1 -> Add/1
  Add/1 -> Inductancce/1
  Inductancce/1 -> Integrator/1
  Inertia/1 -> Integrator1/1
  Kt/1 -> Add1/1
  Add1/1 -> Inertia/1
  Integrator/1 -> Kt/1, Resistance/1
  Voltage/1 -> Add/2
  Dampling/1 -> Add1/2
  Integrator1/1 -> Dampling/1, Speed/1, Ke/1
  Ke/1 -> Add/3

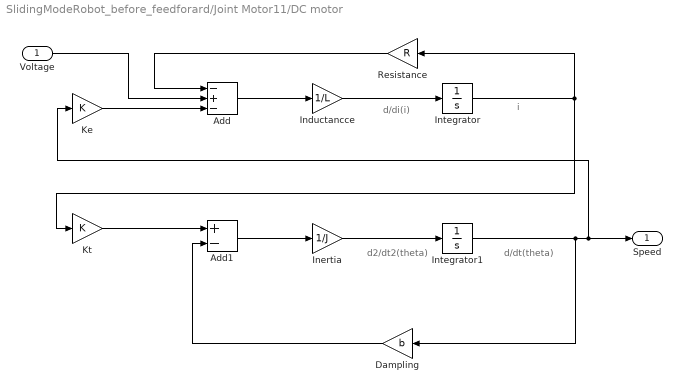
== system SlidingModeRobot_before_feedforard/Joint Motor11/DC motor ==
  note: d/dt(theta)
  note: d2/dt2(theta)
  note: i
  note: d/di(i)
  Voltage : Inport
  Add : Sum  Inputs=-+-
  Add1 : Sum  Inputs=+-
  Dampling : Gain  Gain=b
  Inductancce : Gain  Gain=1/L
  Inertia : Gain  Gain=1/J
  Integrator : Integrator
  Integrator1 : Integrator
  Ke : Gain  Gain=K
  Kt : Gain  Gain=K
  Resistance : Gain  Gain=R
  Speed : Outport
  wires:
  Resistance/1 -> Add/1
  Add/1 -> Inductancce/1
  Inductancce/1 -> Integrator/1
  Inertia/1 -> Integrator1/1
  Kt/1 -> Add1/1
  Add1/1 -> Inertia/1
  Integrator/1 -> Kt/1, Resistance/1
  Voltage/1 -> Add/2
  Dampling/1 -> Add1/2
  Integrator1/1 -> Dampling/1, Speed/1, Ke/1
  Ke/1 -> Add/3

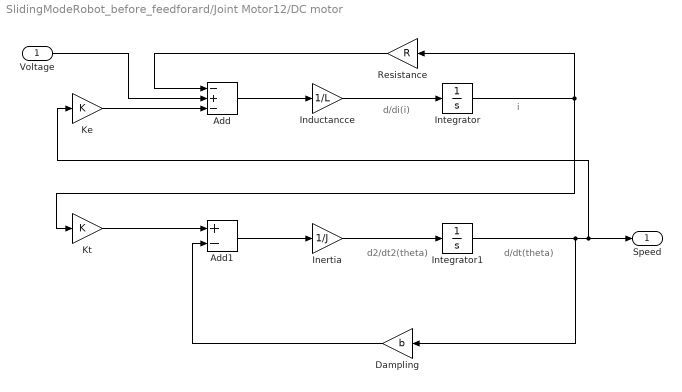
== system SlidingModeRobot_before_feedforard/Joint Motor12/DC motor ==
  note: d/dt(theta)
  note: d2/dt2(theta)
  note: i
  note: d/di(i)
  Voltage : Inport
  Add : Sum  Inputs=-+-
  Add1 : Sum  Inputs=+-
  Dampling : Gain  Gain=b
  Inductancce : Gain  Gain=1/L
  Inertia : Gain  Gain=1/J
  Integrator : Integrator
  Integrator1 : Integrator
  Ke : Gain  Gain=K
  Kt : Gain  Gain=K
  Resistance : Gain  Gain=R
  Speed : Outport
  wires:
  Resistance/1 -> Add/1
  Add/1 -> Inductancce/1
  Inductancce/1 -> Integrator/1
  Inertia/1 -> Integrator1/1
  Kt/1 -> Add1/1
  Add1/1 -> Inertia/1
  Integrator/1 -> Kt/1, Resistance/1
  Voltage/1 -> Add/2
  Dampling/1 -> Add1/2
  Integrator1/1 -> Dampling/1, Speed/1, Ke/1
  Ke/1 -> Add/3

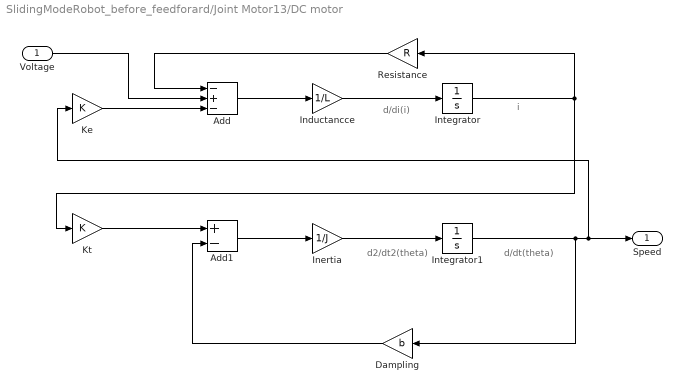
== system SlidingModeRobot_before_feedforard/Joint Motor13/DC motor ==
  note: d/dt(theta)
  note: d2/dt2(theta)
  note: i
  note: d/di(i)
  Voltage : Inport
  Add : Sum  Inputs=-+-
  Add1 : Sum  Inputs=+-
  Dampling : Gain  Gain=b
  Inductancce : Gain  Gain=1/L
  Inertia : Gain  Gain=1/J
  Integrator : Integrator
  Integrator1 : Integrator
  Ke : Gain  Gain=K
  Kt : Gain  Gain=K
  Resistance : Gain  Gain=R
  Speed : Outport
  wires:
  Resistance/1 -> Add/1
  Add/1 -> Inductancce/1
  Inductancce/1 -> Integrator/1
  Inertia/1 -> Integrator1/1
  Kt/1 -> Add1/1
  Add1/1 -> Inertia/1
  Integrator/1 -> Kt/1, Resistance/1
  Voltage/1 -> Add/2
  Dampling/1 -> Add1/2
  Integrator1/1 -> Dampling/1, Speed/1, Ke/1
  Ke/1 -> Add/3

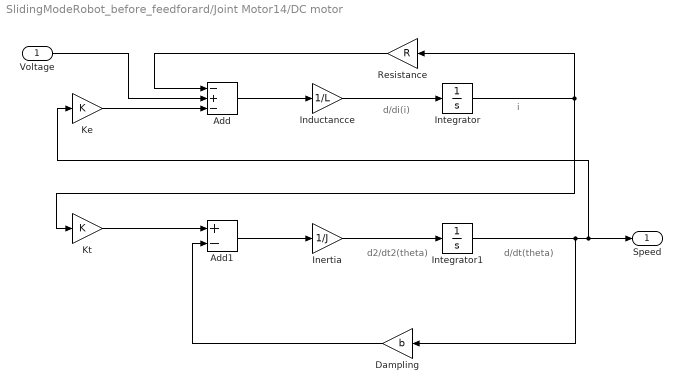
== system SlidingModeRobot_before_feedforard/Joint Motor14/DC motor ==
  note: d/dt(theta)
  note: d2/dt2(theta)
  note: i
  note: d/di(i)
  Voltage : Inport
  Add : Sum  Inputs=-+-
  Add1 : Sum  Inputs=+-
  Dampling : Gain  Gain=b
  Inductancce : Gain  Gain=1/L
  Inertia : Gain  Gain=1/J
  Integrator : Integrator
  Integrator1 : Integrator
  Ke : Gain  Gain=K
  Kt : Gain  Gain=K
  Resistance : Gain  Gain=R
  Speed : Outport
  wires:
  Resistance/1 -> Add/1
  Add/1 -> Inductancce/1
  Inductancce/1 -> Integrator/1
  Inertia/1 -> Integrator1/1
  Kt/1 -> Add1/1
  Add1/1 -> Inertia/1
  Integrator/1 -> Kt/1, Resistance/1
  Voltage/1 -> Add/2
  Dampling/1 -> Add1/2
  Integrator1/1 -> Dampling/1, Speed/1, Ke/1
  Ke/1 -> Add/3

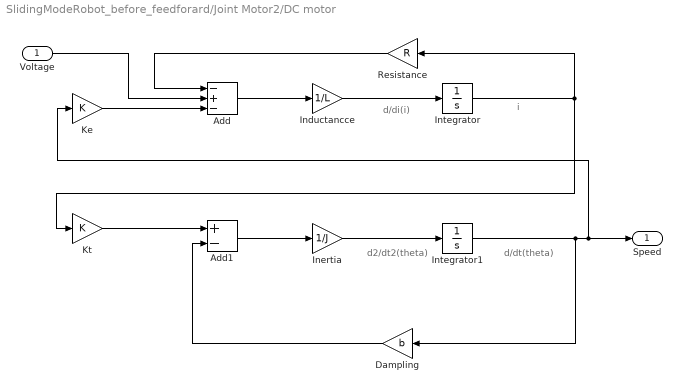
== system SlidingModeRobot_before_feedforard/Joint Motor2/DC motor ==
  note: d/dt(theta)
  note: d2/dt2(theta)
  note: i
  note: d/di(i)
  Voltage : Inport
  Add : Sum  Inputs=-+-
  Add1 : Sum  Inputs=+-
  Dampling : Gain  Gain=b
  Inductancce : Gain  Gain=1/L
  Inertia : Gain  Gain=1/J
  Integrator : Integrator
  Integrator1 : Integrator
  Ke : Gain  Gain=K
  Kt : Gain  Gain=K
  Resistance : Gain  Gain=R
  Speed : Outport
  wires:
  Resistance/1 -> Add/1
  Add/1 -> Inductancce/1
  Inductancce/1 -> Integrator/1
  Inertia/1 -> Integrator1/1
  Kt/1 -> Add1/1
  Add1/1 -> Inertia/1
  Integrator/1 -> Kt/1, Resistance/1
  Voltage/1 -> Add/2
  Dampling/1 -> Add1/2
  Integrator1/1 -> Dampling/1, Speed/1, Ke/1
  Ke/1 -> Add/3

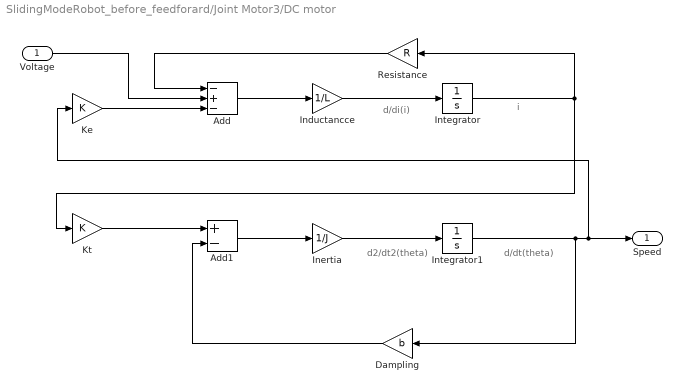
== system SlidingModeRobot_before_feedforard/Joint Motor3/DC motor ==
  note: d/dt(theta)
  note: d2/dt2(theta)
  note: i
  note: d/di(i)
  Voltage : Inport
  Add : Sum  Inputs=-+-
  Add1 : Sum  Inputs=+-
  Dampling : Gain  Gain=b
  Inductancce : Gain  Gain=1/L
  Inertia : Gain  Gain=1/J
  Integrator : Integrator
  Integrator1 : Integrator
  Ke : Gain  Gain=K
  Kt : Gain  Gain=K
  Resistance : Gain  Gain=R
  Speed : Outport
  wires:
  Resistance/1 -> Add/1
  Add/1 -> Inductancce/1
  Inductancce/1 -> Integrator/1
  Inertia/1 -> Integrator1/1
  Kt/1 -> Add1/1
  Add1/1 -> Inertia/1
  Integrator/1 -> Kt/1, Resistance/1
  Voltage/1 -> Add/2
  Dampling/1 -> Add1/2
  Integrator1/1 -> Dampling/1, Speed/1, Ke/1
  Ke/1 -> Add/3

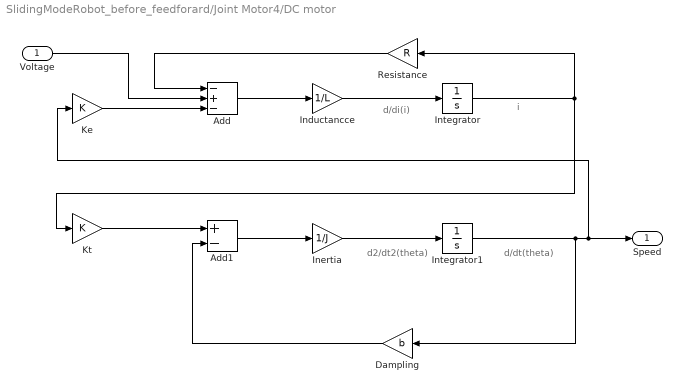
== system SlidingModeRobot_before_feedforard/Joint Motor4/DC motor ==
  note: d/dt(theta)
  note: d2/dt2(theta)
  note: i
  note: d/di(i)
  Voltage : Inport
  Add : Sum  Inputs=-+-
  Add1 : Sum  Inputs=+-
  Dampling : Gain  Gain=b
  Inductancce : Gain  Gain=1/L
  Inertia : Gain  Gain=1/J
  Integrator : Integrator
  Integrator1 : Integrator
  Ke : Gain  Gain=K
  Kt : Gain  Gain=K
  Resistance : Gain  Gain=R
  Speed : Outport
  wires:
  Resistance/1 -> Add/1
  Add/1 -> Inductancce/1
  Inductancce/1 -> Integrator/1
  Inertia/1 -> Integrator1/1
  Kt/1 -> Add1/1
  Add1/1 -> Inertia/1
  Integrator/1 -> Kt/1, Resistance/1
  Voltage/1 -> Add/2
  Dampling/1 -> Add1/2
  Integrator1/1 -> Dampling/1, Speed/1, Ke/1
  Ke/1 -> Add/3

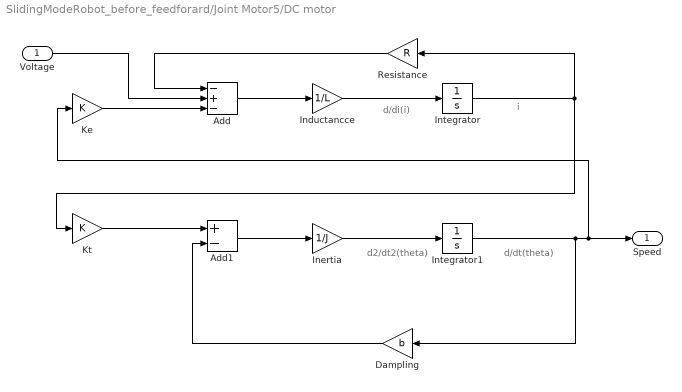
== system SlidingModeRobot_before_feedforard/Joint Motor5/DC motor ==
  note: d/dt(theta)
  note: d2/dt2(theta)
  note: i
  note: d/di(i)
  Voltage : Inport
  Add : Sum  Inputs=-+-
  Add1 : Sum  Inputs=+-
  Dampling : Gain  Gain=b
  Inductancce : Gain  Gain=1/L
  Inertia : Gain  Gain=1/J
  Integrator : Integrator
  Integrator1 : Integrator
  Ke : Gain  Gain=K
  Kt : Gain  Gain=K
  Resistance : Gain  Gain=R
  Speed : Outport
  wires:
  Resistance/1 -> Add/1
  Add/1 -> Inductancce/1
  Inductancce/1 -> Integrator/1
  Inertia/1 -> Integrator1/1
  Kt/1 -> Add1/1
  Add1/1 -> Inertia/1
  Integrator/1 -> Kt/1, Resistance/1
  Voltage/1 -> Add/2
  Dampling/1 -> Add1/2
  Integrator1/1 -> Dampling/1, Speed/1, Ke/1
  Ke/1 -> Add/3

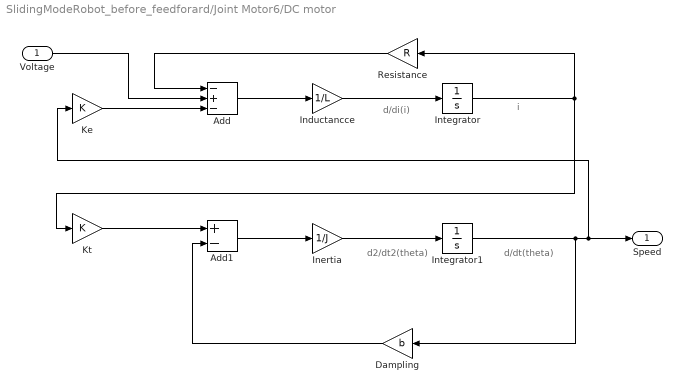
== system SlidingModeRobot_before_feedforard/Joint Motor6/DC motor ==
  note: d/dt(theta)
  note: d2/dt2(theta)
  note: i
  note: d/di(i)
  Voltage : Inport
  Add : Sum  Inputs=-+-
  Add1 : Sum  Inputs=+-
  Dampling : Gain  Gain=b
  Inductancce : Gain  Gain=1/L
  Inertia : Gain  Gain=1/J
  Integrator : Integrator
  Integrator1 : Integrator
  Ke : Gain  Gain=K
  Kt : Gain  Gain=K
  Resistance : Gain  Gain=R
  Speed : Outport
  wires:
  Resistance/1 -> Add/1
  Add/1 -> Inductancce/1
  Inductancce/1 -> Integrator/1
  Inertia/1 -> Integrator1/1
  Kt/1 -> Add1/1
  Add1/1 -> Inertia/1
  Integrator/1 -> Kt/1, Resistance/1
  Voltage/1 -> Add/2
  Dampling/1 -> Add1/2
  Integrator1/1 -> Dampling/1, Speed/1, Ke/1
  Ke/1 -> Add/3

== system SlidingModeRobot_before_feedforard/Joint Motor7/DC motor ==
  note: d/dt(theta)
  note: d2/dt2(theta)
  note: i
  note: d/di(i)
  Voltage : Inport
  Add : Sum  Inputs=-+-
  Add1 : Sum  Inputs=+-
  Dampling : Gain  Gain=b
  Inductancce : Gain  Gain=1/L
  Inertia : Gain  Gain=1/J
  Integrator : Integrator
  Integrator1 : Integrator
  Ke : Gain  Gain=K
  Kt : Gain  Gain=K
  Resistance : Gain  Gain=R
  Speed : Outport
  wires:
  Resistance/1 -> Add/1
  Add/1 -> Inductancce/1
  Inductancce/1 -> Integrator/1
  Inertia/1 -> Integrator1/1
  Kt/1 -> Add1/1
  Add1/1 -> Inertia/1
  Integrator/1 -> Kt/1, Resistance/1
  Voltage/1 -> Add/2
  Dampling/1 -> Add1/2
  Integrator1/1 -> Dampling/1, Speed/1, Ke/1
  Ke/1 -> Add/3

== system SlidingModeRobot_before_feedforard/Joint Motor8/DC motor ==
  note: d/dt(theta)
  note: d2/dt2(theta)
  note: i
  note: d/di(i)
  Voltage : Inport
  Add : Sum  Inputs=-+-
  Add1 : Sum  Inputs=+-
  Dampling : Gain  Gain=b
  Inductancce : Gain  Gain=1/L
  Inertia : Gain  Gain=1/J
  Integrator : Integrator
  Integrator1 : Integrator
  Ke : Gain  Gain=K
  Kt : Gain  Gain=K
  Resistance : Gain  Gain=R
  Speed : Outport
  wires:
  Resistance/1 -> Add/1
  Add/1 -> Inductancce/1
  Inductancce/1 -> Integrator/1
  Inertia/1 -> Integrator1/1
  Kt/1 -> Add1/1
  Add1/1 -> Inertia/1
  Integrator/1 -> Kt/1, Resistance/1
  Voltage/1 -> Add/2
  Dampling/1 -> Add1/2
  Integrator1/1 -> Dampling/1, Speed/1, Ke/1
  Ke/1 -> Add/3

== system SlidingModeRobot_before_feedforard/Joint Motor9/DC motor ==
  note: d/dt(theta)
  note: d2/dt2(theta)
  note: i
  note: d/di(i)
  Voltage : Inport
  Add : Sum  Inputs=-+-
  Add1 : Sum  Inputs=+-
  Dampling : Gain  Gain=b
  Inductancce : Gain  Gain=1/L
  Inertia : Gain  Gain=1/J
  Integrator : Integrator
  Integrator1 : Integrator
  Ke : Gain  Gain=K
  Kt : Gain  Gain=K
  Resistance : Gain  Gain=R
  Speed : Outport
  wires:
  Resistance/1 -> Add/1
  Add/1 -> Inductancce/1
  Inductancce/1 -> Integrator/1
  Inertia/1 -> Integrator1/1
  Kt/1 -> Add1/1
  Add1/1 -> Inertia/1
  Integrator/1 -> Kt/1, Resistance/1
  Voltage/1 -> Add/2
  Dampling/1 -> Add1/2
  Integrator1/1 -> Dampling/1, Speed/1, Ke/1
  Ke/1 -> Add/3
